simulink model "readArray1Timing"  (R2012b)
settings: Solver=FixedStepDiscrete  SolverMode=MultiTasking  StartTime=0.0  StopTime=10.0  FixedStep=0.001  RelTol=1e-3
undefined symbols (not defined in the file): macaddr, modelConstants, rereferencingType
libraries: xpcnetworkbufferlib x4, xpcethernetlib x3, simulink x1
settings Model: xpc_rtwmakecfg_data=_xpcetherlib__xpcether8255xlib__xpcetherGbElib__xpcnblib_  BufferReuse=off  Creator=gilja  LastModifiedBy=Chethan
settings SolverCC: EnableConcurrentExecution=on  ConcurrentTasks=on
settings DataIOCC: SaveOutput=off  SignalLogging=off  DSMLogging=off  SaveTime=off
settings OptimizationCC: BlockReduction=off  InlineParams=on  InlineInvariantSignals=on  OptimizeBlockIOStorage=off  BufferReuse=off  ExpressionFolding=off  LocalBlockOutputs=off
settings HardwareCC: ProdIntDivRoundTo=Zero  ProdEndianess=LittleEndian  ProdHWDeviceType=Generic->32-bit x86 compatible
settings ModelReferenceCC: ModelReferenceNumInstancesAllowed=Single  PropagateVarSize=During execution  ModelReferenceMinAlgLoopOccurrences=on
settings RTWCC: SystemTargetFile=xpctarget.tlc  TemplateMakefile=xpc_default_tmf  Description=xPC Target  ProcessScript=xpctarget_make_rtw_hook  RTWCompilerOptimization=On
settings CodeAppCC: MaxIdLength=62
settings xpcTargetCC: TargetFcnLib=ansi_tfl_table_tmw.mat  CodeReplacementLibrary=XPC_BLAS  ParMdlRefBuildCompliant=on  ConcurrentExecutionCompliant=on  CombineSignalStateStructs=off  GRTInterface=on  xPCTaskExecutionProfile=on  xPCRL32EventNumber=5000  xPCisDownloadable=off  xPCLoadParamSetFile=off  xPCConcurrentTasks=off  xPCEnableSFAnimation=off

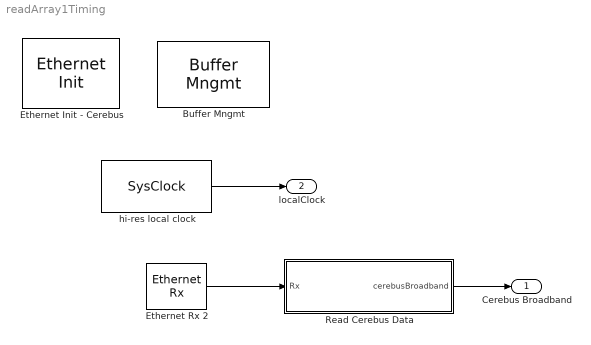
== system readArray1Timing ==
  "Buffer Mngmt " : xpcnetworkbufferlib/Buffer Mngmt   Priority=-1  SampleTime=-1  PoolSizes=[8196 512 4096 65535]  ShowTune=on
  Ethernet Init - Cerebus : xpcethernetlib/Ethernet Init   Priority=-1  ID=1  Driver=Intel Gigabit  Bus=modelConstants.xpcNICConfig.nsp1.bus  Slot=modelConstants.xpcNICConfig.nsp1.slot  SampleTime=-1  AddressSource=Specify  MAC=macaddr('00:00:00:00:00:00')  TxSA=off  RxPromiscuous=off  Multicast={}  RxBad=off  RxShort=off  MaxMTU=1518  TxThreshold=10  TxBuffers=128  RxBuffers=64  ShowTune=on  NumRxBlks=1
  Ethernet Rx 2 : xpcethernetlib/Ethernet Rx   ID=1  SampleTime=modelConstants.sampleTime  Criteria=Receive all unmatched types [0 to 65535]  EtherType=[hex2dec('0000')]  BlkID=0
  Read Cerebus Data : Subsystem
  hi-res local clock : S-Function  InitFcn=try, set_param(gcb,'FunctionName','SysClock'), end  FunctionName=SysClock  SFunctionModules=SysClock_wrapper  EnableBusSupport=off  mask(S-Function Builder){}
      mask help: Simulink:masks:SFunctionBuilder_MD
      mask init:
      | val = [[.9  0.75 0.75 1 1 .9 .9 1]',[1 1 0.75 0.75 .9 .9 1 .9]'];try , sys = get_param(gcb,'SfunBuilderFcnName');if isempty(sys), sys = get_param(gcb,'FunctionName'); end,catch, sys = get_param(gcb,'FunctionName'); end
      settings: CopyFcn=set_param(gcbh,'LinkStatus','none')  PreSaveFcn=try, set_param(gcb,'FunctionName','SysClock'), end  OpenFcn=sfunctionwizard(gcbh)
      mask Display: plot(val(:,1),val(:,2)),disp(sys), port_label('output',1,'sysClk')
  Cerebus Broadband : Outport  OutDataTypeStr=Bus: cerebusBroadband  BusOutputAsStruct=on
  localClock : Outport  Port=2  BusOutputAsStruct=on
  wires:
  Ethernet Rx 2/1 -> Read Cerebus Data/1(Rx)
  Read Cerebus Data/1(cerebusBroadband) -> Cerebus Broadband/1
  hi-res local clock/1 -> localClock/1

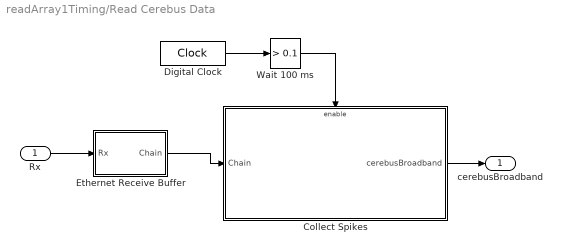
== system readArray1Timing/Read Cerebus Data ==
  Rx : Inport
  Collect Spikes : Subsystem
  Digital Clock : DigitalClock  SampleTime=0.001
  Ethernet Receive Buffer : Subsystem
  Wait 100 ms : simulink/Logic and Bit Operations/Compare To Constant  relop=>  const=0.1  OutDataTypeStr=boolean
  cerebusBroadband : Outport  OutDataTypeStr=Bus: cerebusBroadband
  wires:
  Collect Spikes/1(cerebusBroadband) -> cerebusBroadband/1
  Wait 100 ms/1 -> Collect Spikes/Enable
  Digital Clock/1 -> Wait 100 ms/1
  Ethernet Receive Buffer/1(Chain) -> Collect Spikes/1(Chain)
  Rx/1 -> Ethernet Receive Buffer/1(Rx)

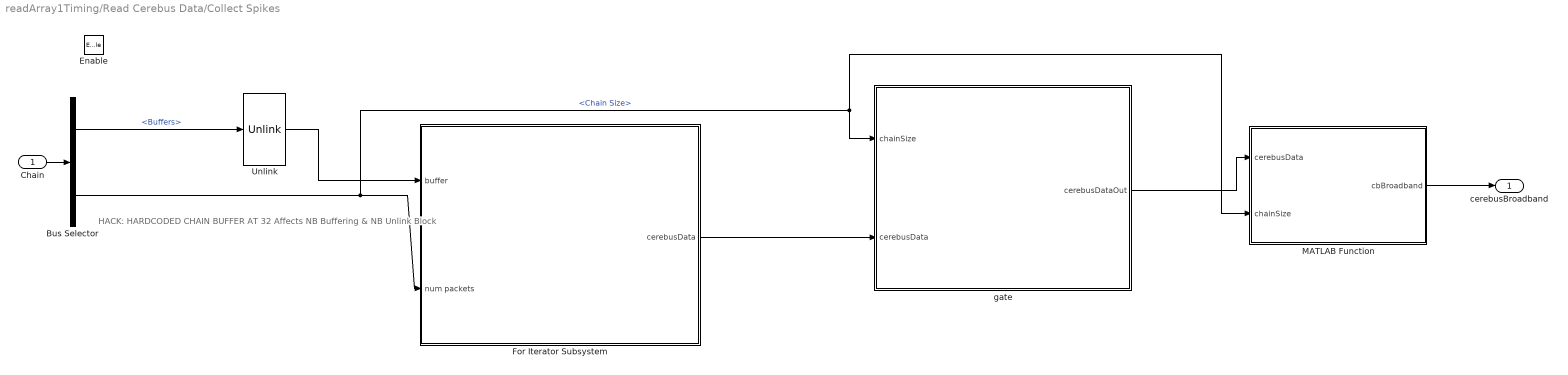
== system readArray1Timing/Read Cerebus Data/Collect Spikes ==
  note: HACK: HARDCODED CHAIN BUFFER AT 32
      | Affects NB Buffering & NB Unlink Block
  Chain : Inport
  Enable : EnablePort  StatesWhenEnabling=reset  PropagateVarSize=During execution
  Bus Selector : BusSelector  OutputSignals=Buffers,Chain Size
  For Iterator Subsystem : Subsystem  TreatAsAtomicUnit=on
  MATLAB Function : MATLAB Function  TreatAsAtomicUnit=on
  "Unlink " : xpcnetworkbufferlib/Unlink   VectorLength=32
  gate : MATLAB Function  TreatAsAtomicUnit=on
  cerebusBroadband : Outport  OutDataTypeStr=Bus: cerebusBroadband
  wires:
  gate/1(cerebusDataOut) -> MATLAB Function/1(cerebusData)
  For Iterator Subsystem/1(cerebusData) -> gate/2(cerebusData)
  Bus Selector/2 -> MATLAB Function/2(chainSize), gate/1(chainSize), For Iterator Subsystem/2(num packets)  "<Chain Size>"
  "Unlink "/1 -> For Iterator Subsystem/1(buffer)
  Bus Selector/1 -> "Unlink "/1  "<Buffers>"
  Chain/1 -> Bus Selector/1
  MATLAB Function/1(cbBroadband) -> cerebusBroadband/1

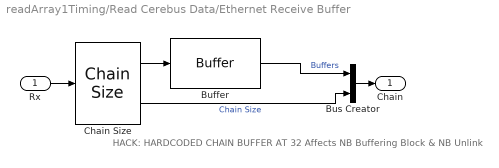
== system readArray1Timing/Read Cerebus Data/Ethernet Receive Buffer ==
  note: HACK: HARDCODED CHAIN BUFFER AT 32
      | Affects NB Buffering Block & NB Unlink
  Rx : Inport
  Buffer : xpcnetworkbufferlib/Buffer   ChainSize=32  BufferSize=0  Threshold=0
  Bus Creator : BusCreator  Inputs=2
  "Chain Size " : xpcnetworkbufferlib/Chain Size 
  Chain : Outport
  wires:
  "Chain Size "/1 -> Buffer/1
  Rx/1 -> "Chain Size "/1
  "Chain Size "/2 -> Bus Creator/2  "Chain Size"
  Bus Creator/1 -> Chain/1
  Buffer/1 -> Bus Creator/1  "Buffers"

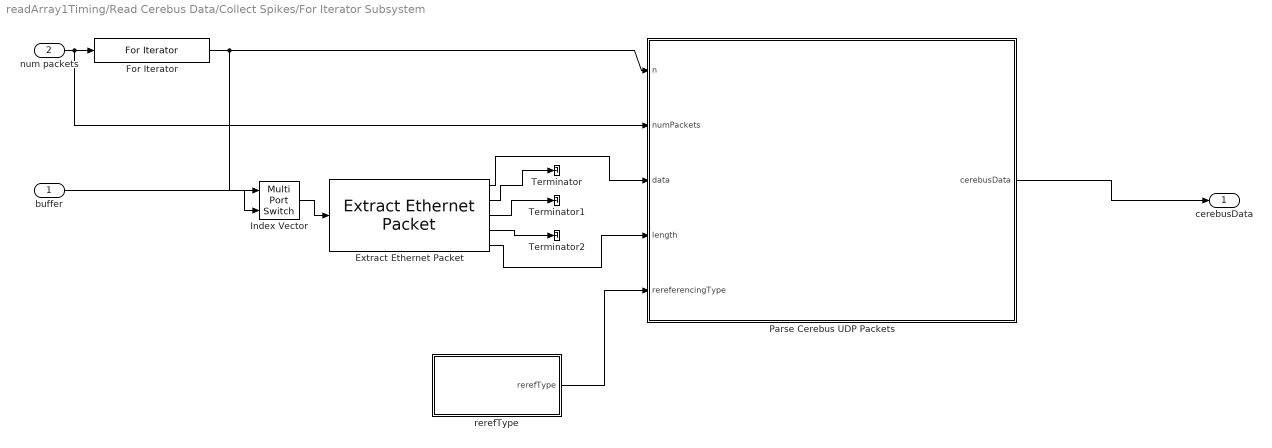
== system readArray1Timing/Read Cerebus Data/Collect Spikes/For Iterator Subsystem ==
  buffer : Inport
  num packets : Inport  Port=2
  Extract Ethernet Packet : xpcethernetlib/Extract Ethernet Packet   EthernetDataSize=1500
  For Iterator : ForIterator  IterationSource=external  IterationVariableDataType=int8
  Index Vector : MultiPortSwitch  Inputs=1
  Parse Cerebus UDP Packets : MATLAB Function  TreatAsAtomicUnit=on
  Terminator : Terminator
  Terminator1 : Terminator
  Terminator2 : Terminator
  rerefType : Subsystem
  cerebusData : Outport  OutDataTypeStr=Bus: cerebusData
  wires:
  Extract Ethernet Packet/4 -> Terminator2/1
  Extract Ethernet Packet/3 -> Terminator1/1
  Extract Ethernet Packet/2 -> Terminator/1
  Parse Cerebus UDP Packets/1(cerebusData) -> cerebusData/1
  Extract Ethernet Packet/1 -> Parse Cerebus UDP Packets/3(data)
  Index Vector/1 -> Extract Ethernet Packet/1
  buffer/1 -> Index Vector/2
  num packets/1 -> Parse Cerebus UDP Packets/2(numPackets), For Iterator/1
  Extract Ethernet Packet/5 -> Parse Cerebus UDP Packets/4(length)
  For Iterator/1 -> Parse Cerebus UDP Packets/1(n), Index Vector/1
  rerefType/1(rerefType) -> Parse Cerebus UDP Packets/5(rereferencingType)

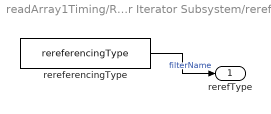
== system readArray1Timing/Read Cerebus Data/Collect Spikes/For Iterator Subsystem/rerefType ==
  rereferencingType : Constant  Value=rereferencingType
  rerefType : Outport
  wires:
  rereferencingType/1 -> rerefType/1  "filterName"

== matlab function readArray1Timing/Read Cerebus Data/Collect Spikes/For Iterator Subsystem/Parse Cerebus UDP Packets ==
  data: n input; numPackets input; data input; cerebusData output Bus: cerebusData; length input; modelConstants parameter; rereferencingType input
function cerebusData = parseBroadbandFromCerebus(n, numPackets, data, length, modelConstants, rereferencingType)
%#codegen 

%%%%%%%%%%%%%%%%%%%%%%%%%%%%%
%
% parse cerebus broadband with common average referencing
%
% Vikash
% Stanford NPTL
% 2/2012
%
%%%%%%%%%%%%%%%%%%%%%%%%%%%%%



%%%%%%%%%%%%%%%%%%%%%%%%%%%%%
% Generic cbPKT data format
%
% values are little endian
%
% uint32 time  // cerebus 30kHz clock
% uint16 chid  // channel id (must be < 0x8000)
% uint8  type
% uint8  dlen  // number of 32-bit (4 byte) data chunks that follows
% *****  data
%%%%%%%%%%%%%%%%%%%%%%%%%%%%%

%%%%%%%%%%%%%%%%%%%%%%%%%%%%%
% cbPKT spike data format
%
% header info: 20 bytes
% spike waveform, max of 128 points (256 bytes)
% internal lab convention of 48 points (96 bytes) results in 1.2 ms data snippet
%
% uint32 time        // cerebus 30kHz clock
% uint16 chid        // channel id (must be 0 < chid < 145)
% uint8  unit        // unit classification (1-5 = sorted unit num, 0 = unclassified, 31 = artifact, 30 = background)
% uint8  dlen        // length of 32-bit (4 byte) data chunks that follows (fixed to 27 for our lab)
% float  fPattern[2] // used for automatic spike sorting
% int16  nPeak       // highest value in spike
% int16  nValley     // lowest values in spike
% int16  wave[48]    // spike waveform
%%%%%%%%%%%%%%%%%%%%%%%%%%%%%



% constants
numCerebusChannels = modelConstants.cerebus.numCerebusChannels;
cerebusIpSource = modelConstants.cerebus.cerebusIpSource;
cerebusIpDest = modelConstants.cerebus.cerebusIpDest;
maxSamplesInMS = modelConstants.cerebus.maxSamplesInMS;

IP_UDP_HEADER_SIZE = uint16(28); % IP header = 20, UDP header = 8

cbPKT_sample_dlen = uint8(numCerebusChannels/2);   

% static variables
% these will contain the final output variables at the end of the for iterator
persistent samplesP;
persistent sampleTimesP;
persistent numSamplesP;

persistent droppedUDPPacketsP;
persistent lastUDPPacketNumberP;

persistent firstCerebusTimeP;
persistent lastCerebusTimeP;

% init persistents
if isempty(droppedUDPPacketsP)
    samplesP = int16(zeros(maxSamplesInMS, numCerebusChannels));
    sampleTimesP = uint32(zeros(maxSamplesInMS,1));
    numSamplesP = uint32(0);
    
    droppedUDPPacketsP = uint32(0);
    lastUDPPacketNumberP = int32(-1);
    
    firstCerebusTimeP = uint32(0);
    lastCerebusTimeP = uint32(0);
end


if n == 1
    samplesP = int16(zeros(maxSamplesInMS, numCerebusChannels));
    numSamplesP = uint32(0);
    sampleTimesP =uint32(zeros(maxSamplesInMS, 1));
end

% Only process packet if it is from cerebus
if(all(data(13:16) == cerebusIpSource') ...
        && all(data(17:20) == cerebusIpDest'))
    
    % yank current packet num in IP header
    udpPacketNumber = int32(data(5))*int32(256) + int32(data(6));
    
    % check for dropped packet
    if(lastUDPPacketNumberP ~= -1)
        droppedUDPPacketsP = droppedUDPPacketsP + uint32(mod(udpPacketNumber-lastUDPPacketNumberP, 2^16) - 1);
    end
    
    lastUDPPacketNumberP = udpPacketNumber;
    
    cbPKT_startpos = uint16(IP_UDP_HEADER_SIZE+1);
    
    firstCbPkt = true;
        
    % parse and copy each spike cbPKT
    while cbPKT_startpos < length
        
        cbPKT_chid_lsb = data(cbPKT_startpos + 4);  % extract channel lsb
        cbPKT_chid_msb = data(cbPKT_startpos + 5);  % extract channel msb
        cbPKT_type = data(cbPKT_startpos + 6);      % extract unit classification
        cbPKT_dlen = data(cbPKT_startpos + 7);      % extract data length of "non header" data
        
        if( (n== 1) && (firstCbPkt) )
            firstCerebusTimeP = uint32(data(cbPKT_startpos))*2^(0*8) + uint32(data(cbPKT_startpos+1))*2^(1*8) + uint32(data(cbPKT_startpos+2))*2^(2*8) + uint32(data(cbPKT_startpos+3))*2^(3*8);
            firstCbPkt = false;
        end
        
        lastCerebusTimeP = uint32(data(cbPKT_startpos))*2^(0*8) + uint32(data(cbPKT_startpos+1))*2^(1*8) + uint32(data(cbPKT_startpos+2))*2^(2*8) + uint32(data(cbPKT_startpos+3))*2^(3*8);
        
        
        % Check for group packet type 5 (broadband, 30 kS/s)    
        if (cbPKT_chid_lsb == 0) && (cbPKT_chid_msb == 0) && ...
                (cbPKT_dlen == cbPKT_sample_dlen) && ...
                (cbPKT_type == 5)
            
            numSamplesP = numSamplesP + 1;
            
            sampleTimesP(numSamplesP) = uint32(data(cbPKT_startpos))*2^(0*8) + uint32(data(cbPKT_startpos+1))*2^(1*8) + uint32(data(cbPKT_startpos+2))*2^(2*8) + uint32(data(cbPKT_startpos+3))*2^(3*8);
            
            for x = coder.unroll(1:numCerebusChannels)
                tmpSample = int32(data(cbPKT_startpos + 8 + 2*x - 2))*(2^(0*8)) + int32(data(cbPKT_startpos + 8 + 2*x - 1))*(2^(1*8));
                if(tmpSample > 2^15)
                    samplesP(numSamplesP, x) = int16(tmpSample - 2^16);
                else
                    samplesP(numSamplesP, x) = int16(tmpSample);
                end
                
            end
            switch rereferencingType
                case rigHardwareConstants.REREFERENCE_COMMON_AVG
                    % Common avg reference:
                    samplesP(numSamplesP, :) = samplesP(numSamplesP, :) - mean(samplesP(numSamplesP, :));
                case rigHardwareConstants.REREFERENCE_COMMON_MEDIAN
                    % Common median reference:
                    samplesP(numSamplesP, :) = samplesP(numSamplesP, :) - int16(median(double(samplesP(numSamplesP, :))));
            end
            
                    
        end
        
        cbPKT_startpos = cbPKT_startpos + uint16(8) + uint16(cbPKT_dlen)*4;
    end
    
    
end

cerebusData.droppedUDPPackets = droppedUDPPacketsP;
cerebusData.lastUDPPacketNumber = lastUDPPacketNumberP;

% update large arrays only at end of for loop
if n == numPackets
    cerebusData.numSamples = numSamplesP;
    cerebusData.samples = samplesP;
    cerebusData.sampleTimes = sampleTimesP;
    
    cerebusData.firstCerebusTime = firstCerebusTimeP;
    cerebusData.lastCerebusTime = lastCerebusTimeP;
else
    cerebusData.numSamples = uint32(0);
    cerebusData.samples = coder.nullcopy(int16(zeros(maxSamplesInMS, numCerebusChannels)));
    cerebusData.sampleTimes = coder.nullcopy(uint32(zeros(maxSamplesInMS,1)));
    
    cerebusData.firstCerebusTime = uint32(0);
    cerebusData.lastCerebusTime = uint32(0);
end

== matlab function readArray1Timing/Read Cerebus Data/Collect Spikes/MATLAB Function ==
  data: cerebusData input Bus: cerebusData; cbBroadband output Bus: cerebusBroadband size=1; modelConstants parameter; chainSize input
function cbBroadband  = bufferCerebusSamples(cerebusData, modelConstants, chainSize)
%#codegen

persistent sampleBuffer bufferInIdx bufferOutIdx outputValidP bufferInit;

numCerebusChannels = modelConstants.cerebus.numCerebusChannels;
bufferSize = modelConstants.cerebus.sampleBufferSize;
bufferDelay = modelConstants.cerebus.sampleBufferDelay;


if(isempty(sampleBuffer))
    sampleBuffer = int16(zeros(bufferSize, numCerebusChannels));
    bufferInIdx = 0;
    bufferOutIdx = bufferSize;
    outputValidP = false;
    bufferInit = true;
end

cerebusFrame = int16(zeros(30, numCerebusChannels));

if(bufferInIdx < bufferOutIdx)
    bufferSpace = bufferOutIdx - bufferInIdx;
else
    bufferSpace = bufferSize - bufferInIdx + bufferOutIdx;
end

if(cerebusData.numSamples > bufferSpace)
    bufferInit = false;
    outputValidP = false;
end

% if((cerebusData.numSamples > 0) && (cerebusData.numSamples < bufferSize))
%     sampleBuffer(bufferInIdx + [1:cerebusData.numSamples], :) = cerebusData.samples(1:cerebusData.numSamples, :);
%     bufferInIdx = mod((bufferInIdx + double(cerebusData.numSamples)), bufferSize);
% end

if((cerebusData.numSamples > 0) && (cerebusData.numSamples < bufferSpace))
    for nn = 1:cerebusData.numSamples
        indx= 1+mod(double(bufferInIdx + nn)-1, bufferSize);
        sampleBuffer(indx, :) = cerebusData.samples(nn, :);
    end
    bufferInIdx = mod((bufferInIdx + double(cerebusData.numSamples)), bufferSize);
end

if(bufferInit)
    if(bufferInIdx >= (bufferDelay))
        bufferInit = false;
        outputValidP = true;
    end
elseif(outputValidP)
    numToEndOfBuffer = bufferSize - bufferOutIdx;
    if( (numToEndOfBuffer >= 30) && ...
            ((bufferInIdx >= bufferOutIdx + 30) || (bufferInIdx < bufferOutIdx)) )
        cerebusFrame = sampleBuffer(bufferOutIdx+[1:30], :);
        
    elseif ( (numToEndOfBuffer < 30) ...
            && (bufferInIdx >= (30 - numToEndOfBuffer) ))
        idx = [1:30];
        idx(1:numToEndOfBuffer) = idx(1:numToEndOfBuffer) + bufferOutIdx;
        idx(numToEndOfBuffer+1:end) = idx(numToEndOfBuffer+1:end) - numToEndOfBuffer;
        cerebusFrame = sampleBuffer(idx, :);
        
    else
        outputValidP = false;
    end
    
    bufferOutIdx = mod((bufferOutIdx + 30), bufferSize);
end

cbBroadband.cerebusFrame = cerebusFrame;
cbBroadband.outputValid = outputValidP;
cbBroadband.numDroppedUDPPackets = cerebusData.droppedUDPPackets;
cbBroadband.chainSize = uint16(chainSize); %% this will be set downstream

== matlab function readArray1Timing/Read Cerebus Data/Collect Spikes/gate ==
  data: chainSize input; cerebusDataOut output Bus: cerebusData; cerebusData input Bus: cerebusData; modelConstants parameter
function cerebusDataOut = checkNoPackets(chainSize, cerebusData, modelConstants)


if chainSize == 0
    cerebusData.samples = coder.nullcopy(int16(zeros(modelConstants.cerebus.maxSamplesInMS, modelConstants.cerebus.numCerebusChannels)));
    cerebusData.sampleTimes = coder.nullcopy(uint32(zeros(modelConstants.cerebus.maxSamplesInMS,1)));
    cerebusData.numSamples = uint32(0);
    
    cerebusData.firstCerebusTime = uint32(0);
    cerebusData.lastCerebusTime = uint32(0);
end

cerebusDataOut = cerebusData;
